simulink model "Matlab Simulink"  (R2023b)
settings: Solver=FixedStepAuto  StartTime=0.0  StopTime=5  FixedStep=0.0001  RelTol=1e-3
libraries: fuzblock x1
settings Model: Creator=Hamid Reza  LastModifiedBy=Hamid Reza

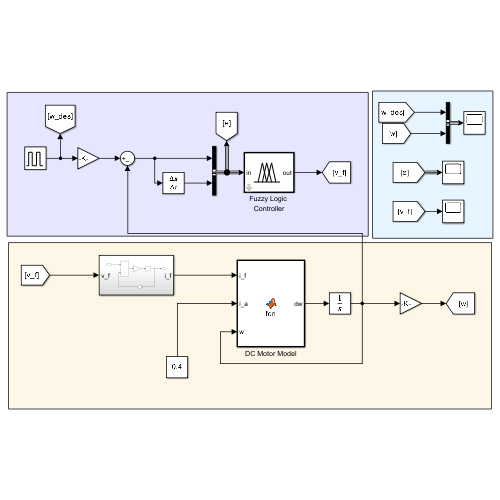
[thumbnail: Simulink's stored preview of the top-level diagram]
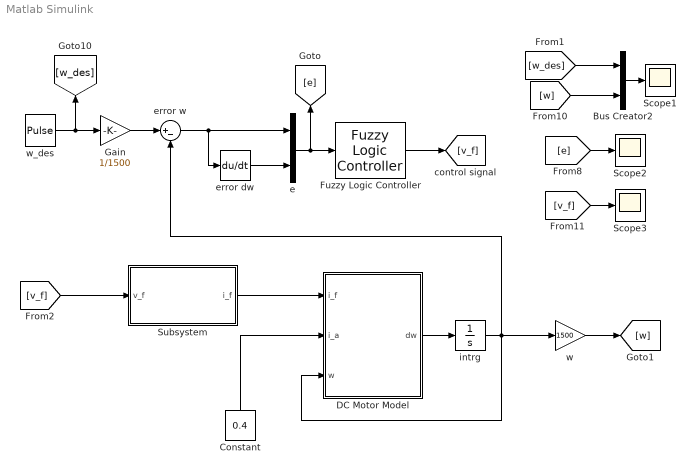
== system Matlab Simulink ==
  Bus Creator2 : BusCreator  Inputs=2
  Constant : Constant  Value=0.4
  DC Motor Model : MATLAB Function  TreatAsAtomicUnit=on
  Fuzzy Logic Controller : fuzblock/Fuzzy Logic  Controller  FIS='custom_controller.fis'  OutputSampleNumber=101  DataType=double  FuzzifiedInputs=off  RuleFiringStrengths=off  RuleOutputs=off  AggregatedOutputs=off  SimulateUsing=Interpreted execution  OutOfRangeInputValueMessage=warning  NoRuleFiredMessage=warning  EmptyOutputFuzzySetMessage=warning
  Gain : Gain  Gain=1/1500
  Scope1 : Scope
  Scope2 : Scope
  Scope3 : Scope
  Subsystem : Subsystem
  e : BusCreator  Inputs=2
  error dw : Derivative
  error w : Sum  Inputs=|+-
  intrg : Integrator
  w : Gain  Gain=1500
  w_des : DiscretePulseGenerator  PulseType=Time based  Amplitude=125  Period=0.5  PulseWidth=50
  wires:
  [e] -> Scope2/1
  [w_des] -> Bus Creator2/1
  [w] -> Bus Creator2/2
  Bus Creator2/1 -> Scope1/1
  [v_f] -> Scope3/1
  Fuzzy Logic Controller/1 -> [v_f]
  Constant/1 -> DC Motor Model/2(i_a)
  Subsystem/1(i_f) -> DC Motor Model/1(i_f)
  [v_f] -> Subsystem/1(v_f)
  DC Motor Model/1(dw) -> intrg/1
  w_des/1 -> Gain/1, [w_des]
  intrg/1 -> w/1, DC Motor Model/3(w), error w/2
  e/1 -> Fuzzy Logic Controller/1, [e]
  error dw/1 -> e/2
  w/1 -> [w]
  Gain/1 -> error w/1
  error w/1 -> error dw/1, e/1

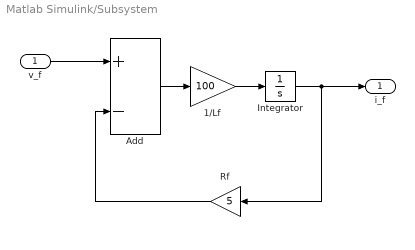
== system Matlab Simulink/Subsystem ==
  v_f : Inport
  1/Lf : Gain  Gain=100
  Add : Sum  Inputs=+-
  Integrator : Integrator
  Rf : Gain  Gain=5
  i_f : Outport
  wires:
  v_f/1 -> Add/1
  Add/1 -> 1/Lf/1
  1/Lf/1 -> Integrator/1
  Integrator/1 -> Rf/1, i_f/1
  Rf/1 -> Add/2

== matlab function Matlab Simulink/DC Motor Model ==
  data: i_f input; i_a input; dw output; w input
function dw = fcn(i_f,i_a, w)

Kt = 0.7;       % Torque Constant
Kf = 0.08;      % Field Constant
j = 0.000162;   % Moment of inertia
Tl = 0.001;     % Load Torque
b = 0.0065;     % Viscous coefficient


dw = ( Kt*Kf*i_f*i_a - b*w - Tl)/j ;
